simulink model "DC_motor_drive_system"  (R2019b)
settings: Solver=VariableStepAuto  StartTime=0.0  StopTime=0.8  RelTol=1e-3
settings Model: Creator=100448597  LastModifiedBy=robom
settings SFSimCC: CustomCodeUndefinedFunction=UseInterfaceOnly

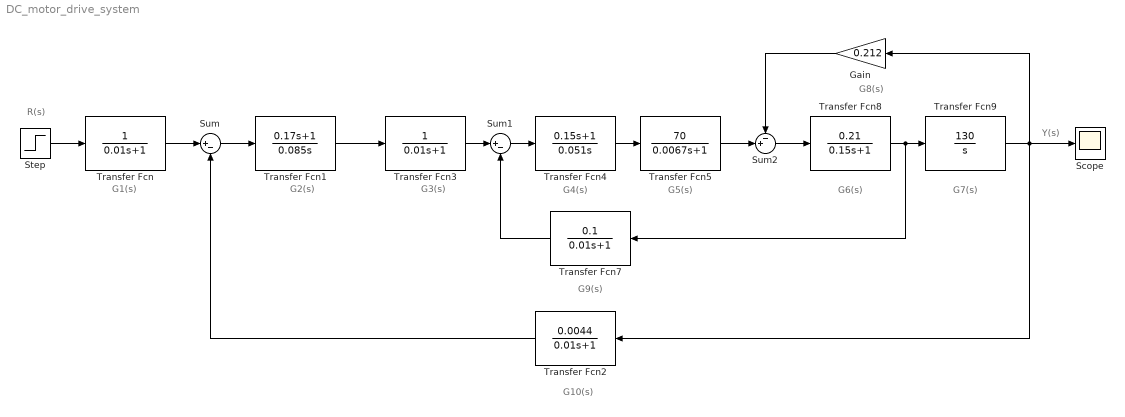
== system DC_motor_drive_system ==
  note: R(s)
  note: G1(s)
  note: G2(s)
  note: G3(s)
  note: G4(s)
  note: G5(s)
  note: G6(s)
  note: G7(s)
  note: G8(s)
  note: G9(s)
  note: G10(s)
  note: Y(s)
  Gain : Gain  Gain=0.212
  Scope : Scope
  Step : Step  Time=0  SampleTime=0
  Sum : Sum  Inputs=|+-
  Sum1 : Sum  Inputs=|+-
  Sum2 : Sum  Inputs=-+|
  Transfer Fcn : TransferFcn  Numerator=1  Denominator=[0.01 1]
  Transfer Fcn1 : TransferFcn  Numerator=[0.17 1]  Denominator=[0.085 0]
  Transfer Fcn2 : TransferFcn  Numerator=0.0044  Denominator=[0.01 1]
  Transfer Fcn3 : TransferFcn  Numerator=1  Denominator=[0.01 1]
  Transfer Fcn4 : TransferFcn  Numerator=[0.15 1]  Denominator=[0.051 0]
  Transfer Fcn5 : TransferFcn  Numerator=70  Denominator=[0.0067 1]
  Transfer Fcn7 : TransferFcn  Numerator=0.1  Denominator=[0.01 1]
  Transfer Fcn8 : TransferFcn  Numerator=0.21  Denominator=[0.15 1]
  Transfer Fcn9 : TransferFcn  Numerator=130  Denominator=[1 0]
  wires:
  Transfer Fcn/1 -> Sum/1
  Sum/1 -> Transfer Fcn1/1
  Step/1 -> Transfer Fcn/1
  Transfer Fcn2/1 -> Sum/2
  Transfer Fcn1/1 -> Transfer Fcn3/1
  Transfer Fcn3/1 -> Sum1/1
  Sum1/1 -> Transfer Fcn4/1
  Transfer Fcn4/1 -> Transfer Fcn5/1
  Transfer Fcn5/1 -> Sum2/2
  Gain/1 -> Sum2/1
  Transfer Fcn7/1 -> Sum1/2
  Sum2/1 -> Transfer Fcn8/1
  Transfer Fcn8/1 -> Transfer Fcn7/1, Transfer Fcn9/1
  Transfer Fcn9/1 -> Scope/1, Gain/1, Transfer Fcn2/1
